simulink model "FSO_Model"  (R2025a)
settings: Solver=VariableStepAuto  StartTime=0.0  StopTime=2  RelTol=1e-3
libraries: simulink x1, commsink2 x1, mcbhdlcontrolslib x1, commrandsrc3 x1
settings Model: Creator=dhruv  LastModifiedBy=dhruv

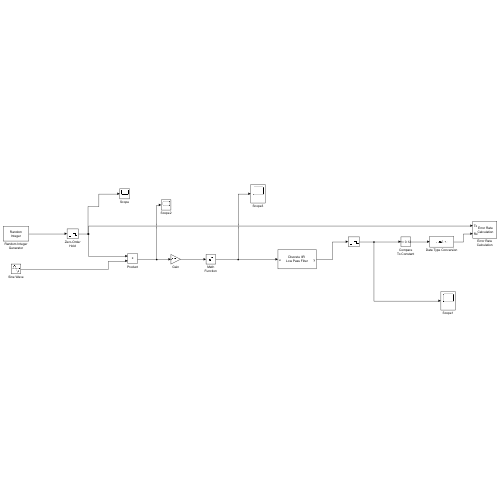
[thumbnail: Simulink's stored preview of the top-level diagram]
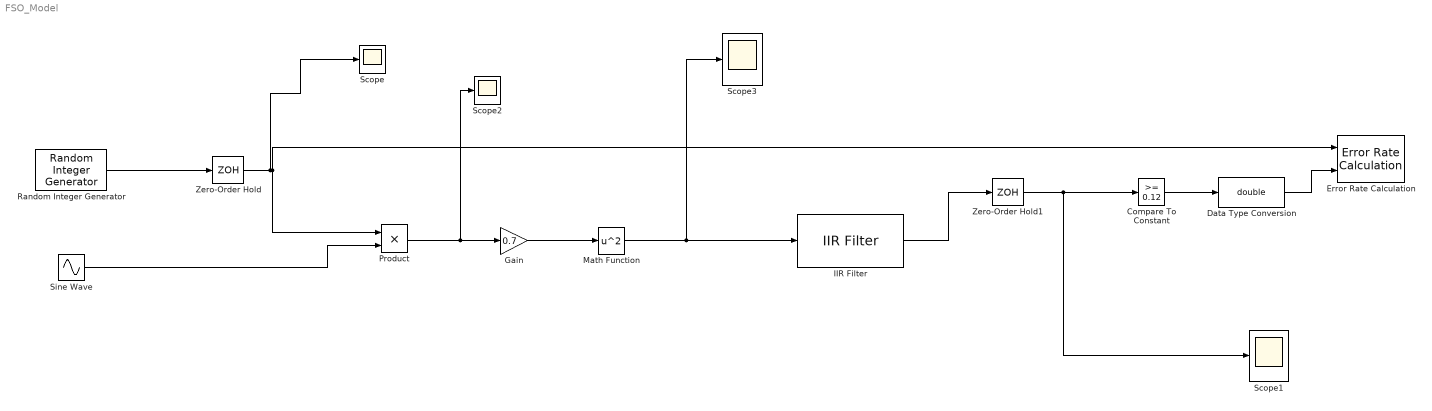
== system FSO_Model ==
  Compare To Constant : simulink/Logic and Bit Operations/Compare To Constant  relop=>=  const=0.12  OutDataTypeStr=boolean
  Data Type Conversion : DataTypeConversion  OutDataTypeStr=double  SaturateOnIntegerOverflow=off  RndMeth=Floor
  Error Rate Calculation : commsink2/Error Rate Calculation  N=0  st_delay=0  cp_mode=Entire frame  subframe=[]  PMode=Workspace  WsName=BER  RsMode2=off  stop=off  numErr=100  maxBits=1e6
      settings: LibrarySourceBlock=|
      | commhdlsink/Error Rate
      | Calculation
  Gain : Gain  Gain=0.7
  IIR Filter : mcbhdlcontrolslib/IIR Filter  VariantControl=Low Pass Filter  VariantSelect=Low-pass  FilterConstantInputType=Specify via dialog  Filter_constant=0.15  advancedSettings=off  Ts=50e-6  cutOff_freq=561.7233
      settings: LibrarySourceBlock=mcbhdllib/Signal Management/IIR Filter
  Math Function : Math  Operator=square
  Product : Product
  Random Integer Generator : commrandsrc3/Random Integer Generator  SetSize=2  SeedSource=Auto  Seed=0  SampleTime=1e-6  SamplesPerFrame=1  OutputDataType=double  SimulateUsing=Interpreted execution
  Scope{,1..3} (4 alike) : Scope
      Scope settings: ActiveDisplayYMinimum=-0.12499999999999997  ActiveDisplayYMaximum=1.125
      Scope1 settings: ActiveDisplayYMinimum=-0.034248714353590969  ActiveDisplayYMaximum=0.30823842918231881
      Scope2 settings: ActiveDisplayYMinimum=-1.1888206453689421  ActiveDisplayYMaximum=1.1888206453689421  DataLoggingVariableName=ScopeData2
      Scope3 settings: ActiveDisplayYMinimum=-0.055401145452732753  ActiveDisplayYMaximum=0.49861030907459492  DataLoggingVariableName=ScopeData3
  Sine Wave : Sin  SineType=Sample based  Frequency=1e-6  SampleTime=1e-6
  Zero-Order Hold : ZeroOrderHold  SampleTime=1e-6
  Zero-Order Hold1 : ZeroOrderHold  SampleTime=1e-6
  wires:
  Random Integer Generator/1 -> Zero-Order Hold/1
  Zero-Order Hold/1 -> Scope/1, Product/1, Error Rate Calculation/1
  Sine Wave/1 -> Product/2
  Product/1 -> Scope2/1, Gain/1
  Gain/1 -> Math Function/1
  Compare To Constant/1 -> Data Type Conversion/1
  Data Type Conversion/1 -> Error Rate Calculation/2
  Math Function/1 -> Scope3/1, IIR Filter/1
  IIR Filter/1 -> Zero-Order Hold1/1
  Zero-Order Hold1/1 -> Scope1/1, Compare To Constant/1
